simulink model "Loops1"  (Simulink 6.0)
settings: Solver=ode45  StartTime=0.0  StopTime=10.0  RelTol=1e-3
settings Model: Creator=scaife  LastModifiedBy=scaife  ExtModeAutoUpdateStatusClock=off
settings DataIOCC: SignalLoggingName=sigsOut
settings DebuggingCC: SolverPrmCheckMsg=none
settings HardwareCC: TargetUnknown=on
settings GRTTargetCC: ModelReferenceCompliant=off  MatFileLogging=off

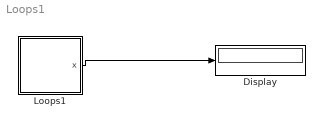
== system Loops1 ==
  Display : Display
  Loops1 : Stateflow chart
  wires:
  Loops1/1(x) -> Display/1

== stateflow chart Loops1 ==
  state A
  state B
  A -> (junction 5) : {x=0}
  (junction 5) -> B
  (default) -> A
  (junction 5) -> (junction 5) : [x<2]{x++}
  B -> A
  data: x output int32
